simulink model "dir_sim"  (R2017b)
settings: Solver=VariableStepAuto  StartTime=0.0  StopTime=5  RelTol=1e-3
settings Model: Creator=Administrator  LastModifiedBy=Administrator
settings SolverCC: AlgebraicLoopSolver=LineSearch

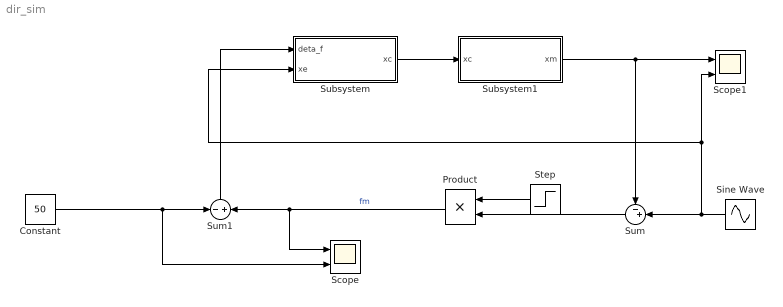
== system dir_sim ==
  Constant : Constant  Value=50
  Product : Product
  Scope : Scope  NumInputPorts=2
  Scope1 : Scope  NumInputPorts=2
  Sine Wave : Sin  SampleTime=0
  Step : Step  Time=3  Before=2000  After=3000  SampleTime=0
  Subsystem : Subsystem
  Subsystem1 : Subsystem
  Sum : Sum  Inputs=-+|
  Sum1 : Sum  Inputs=-|+
  wires:
  Sine Wave/1 -> Subsystem/2(xe), Scope1/2, Sum/2
  Subsystem/1(xc) -> Subsystem1/1(xc)
  Constant/1 -> Scope/2, Sum1/1
  Sum1/1 -> Subsystem/1(deta_f)
  Sum/1 -> Product/2
  Step/1 -> Product/1
  Product/1 -> Scope/1, Sum1/2  "fm"
  Subsystem1/1(xm) -> Sum/1, Scope1/1

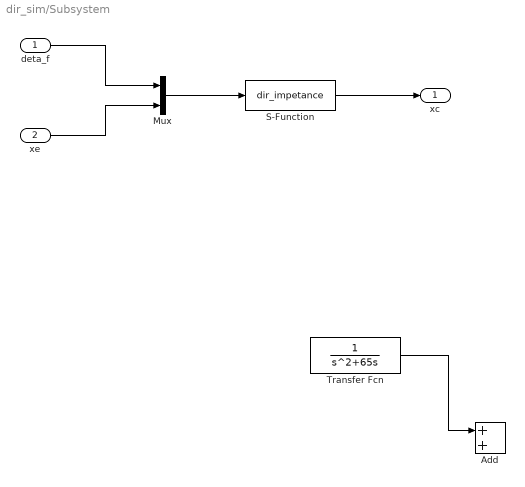
== system dir_sim/Subsystem ==
  deta_f : Inport
  xe : Inport  Port=2
  Add : Sum
  Mux : Mux  Inputs=2
  S-Function : S-Function  FunctionName=dir_impetance  SFunctionDeploymentMode=off  EnableBusSupport=off
  Transfer Fcn : TransferFcn  Denominator=[1 65 0]
  xc : Outport
  wires:
  Mux/1 -> S-Function/1
  Transfer Fcn/1 -> Add/1
  S-Function/1 -> xc/1
  deta_f/1 -> Mux/1
  xe/1 -> Mux/2

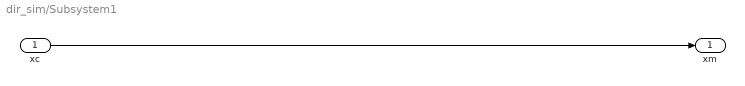
== system dir_sim/Subsystem1 ==
  xc : Inport
  xm : Outport
  wires:
  xc/1 -> xm/1
